simulink model "Signal4"  (Simulink 9.1)
settings: Solver=ode45  StartTime=0.0  StopTime=20  RelTol=1e-3  EnableMultiTasking=on
settings Model: Creator=Admin  LastModifiedBy=Asus
settings DataIOCC: LimitDataPoints=on  SignalLoggingSaveFormat=ModelDataLogs
settings OptimizationCC: ExpressionDepthLimit=2147483647
settings DebuggingCC: SolverPrmCheckMsg=warning  FcnCallInpInsideContextMsg=warning  StateNameClashWarn=warning
settings GRTTargetCC: GeneratePreprocessorConditionals=Disable all  CombineOutputUpdateFcns=on  GRTInterface=off

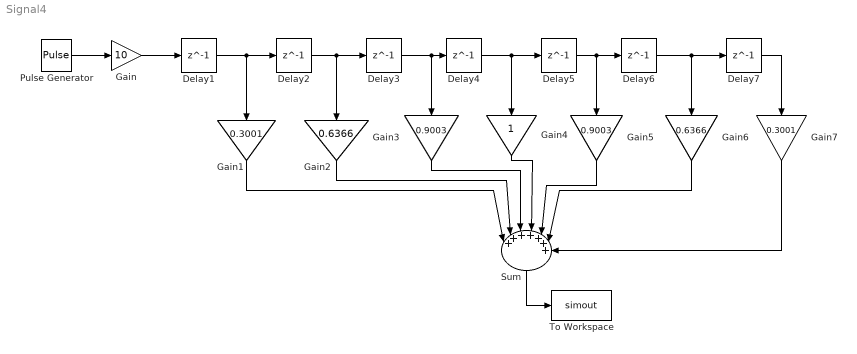
== system Signal4 ==
  Delay{1..7} (7 alike) : Delay  DelayLength=1
  Gain : Gain  Gain=10
  Gain1 : Gain  Gain=0.3001
  Gain2 : Gain  Gain=0.6366
  Gain3 : Gain  Gain=0.9003
  Gain4 : Gain
  Gain5 : Gain  Gain=0.9003
  Gain6 : Gain  Gain=0.6366
  Gain7 : Gain  Gain=0.3001
  Pulse Generator : DiscretePulseGenerator  Period=100
  Sum : Sum  Inputs=|+++++++
  To Workspace : ToWorkspace  VariableName=simout  SampleTime=-1
  wires:
  Pulse Generator/1 -> Gain/1
  Gain/1 -> Delay1/1
  Delay1/1 -> Delay2/1, Gain1/1
  Delay2/1 -> Delay3/1, Gain2/1
  Delay3/1 -> Delay4/1, Gain3/1
  Delay4/1 -> Delay5/1, Gain4/1
  Delay5/1 -> Delay6/1, Gain5/1
  Delay6/1 -> Delay7/1, Gain6/1
  Delay7/1 -> Gain7/1
  Gain1/1 -> Sum/1
  Gain2/1 -> Sum/2
  Gain3/1 -> Sum/3
  Gain4/1 -> Sum/4
  Gain5/1 -> Sum/5
  Gain6/1 -> Sum/6
  Gain7/1 -> Sum/7
  Sum/1 -> To Workspace/1
